simulink model "avr_simulation"  (R2021b)
settings: Solver=VariableStepAuto  StartTime=0.0  StopTime=1  RelTol=1e-3
undefined symbols (not defined in the file): E_1, E_2, initialOffset2, S_E_E1, S_E_E2, Ts
libraries: simulink x8, eeGeneralControl x6
settings Model: Creator=mouht  LastModifiedBy=mouht

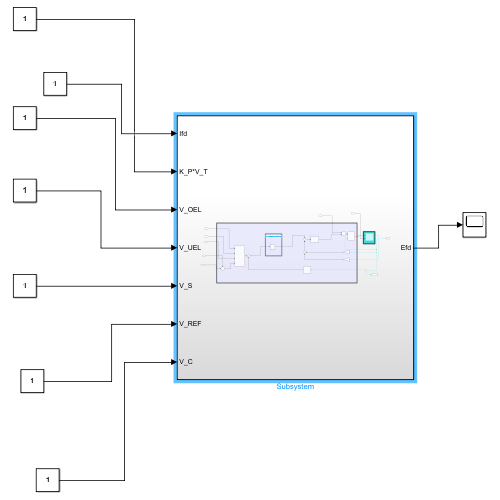
[thumbnail: Simulink's stored preview of the top-level diagram]
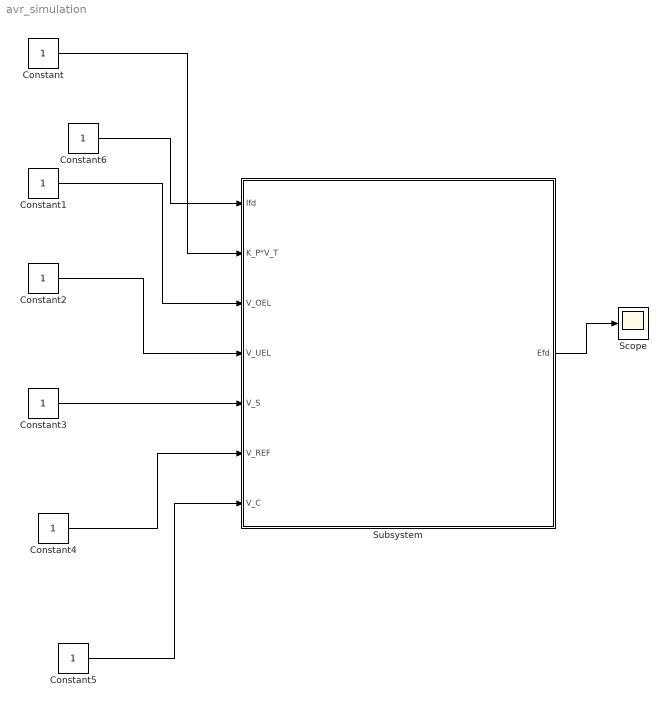
== system avr_simulation ==
  Constant{,1..6} (7 alike) : Constant
  Scope : Scope
  Subsystem : Subsystem
  wires:
  Constant5/1 -> Subsystem/7("V_C ")
  Constant4/1 -> Subsystem/6(V_REF)
  Constant3/1 -> Subsystem/5(V_S)
  Constant2/1 -> Subsystem/4(V_UEL)
  Constant1/1 -> Subsystem/3(V_OEL)
  Constant/1 -> Subsystem/2(K_P*V_T)
  Constant6/1 -> Subsystem/1(Ifd)
  Subsystem/1(Efd) -> Scope/1

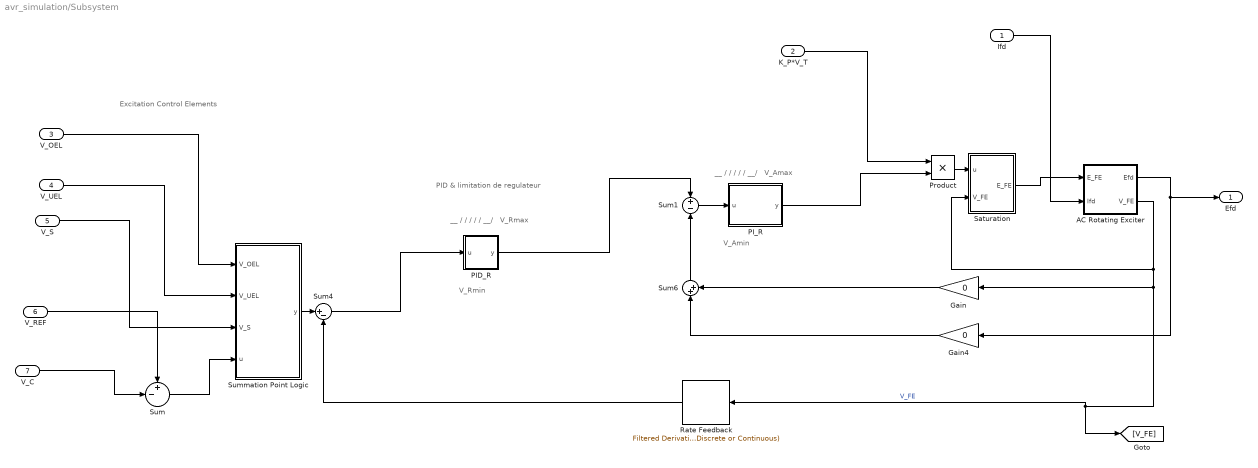
== system avr_simulation/Subsystem ==
  note: PID & limitation de regulateur
  note: __
      |               /
      |             /
      |           /
      |         /
      |       /
      | __/
  note: Excitation
      | Control
      | Elements
  note: V_Rmax
  note: V_Rmin
  note: __
      |               /
      |             /
      |           /
      |         /
      |       /
      | __/
  note: V_Amax
  note: V_Amin
  Ifd : Inport
  K_P*V_T : Inport  Port=2
  V_OEL : Inport  Port=3
  V_UEL : Inport  Port=4
  V_S : Inport  Port=5
  V_REF : Inport  Port=6
  "V_C " : Inport  Port=7
  AC Rotating Exciter : Subsystem
  Gain : Gain  Gain=0
  Gain4 : Gain  Gain=0
  PID_R : Subsystem
  PI_R : Subsystem
  Product : Product
  Rate Feedback : eeGeneralControl/Filtered Derivative (Discrete or Continuous)  K=0  T=1  B=inf  A=-inf  minRatio=10  init_option=Inherited from block input  x0=0  Ts=-1
      settings: SourceProductBaseCode=PS
  Saturation : Subsystem
  Sum : Sum  Inputs=+-|  InputSameDT=on  SaturateOnIntegerOverflow=on  OutDataTypeStr=Inherit: Same as first input
  Sum1 : Sum  Inputs=+-  InputSameDT=on  SaturateOnIntegerOverflow=on  OutDataTypeStr=Inherit: Same as first input
  Sum4 : Sum  Inputs=|+-  InputSameDT=on  SaturateOnIntegerOverflow=on  OutDataTypeStr=Inherit: Same as first input
  Sum6 : Sum  Inputs=|++  InputSameDT=on  SaturateOnIntegerOverflow=on  OutDataTypeStr=Inherit: Same as first input
  Summation Point Logic : Subsystem
  Efd : Outport
  wires:
  Product/1 -> Saturation/1(u)
  AC Rotating Exciter/2(V_FE) -> [V_FE], Rate Feedback/1, Gain/1, Saturation/2(V_FE)  "V_FE"
  Gain/1 -> Sum6/2
  Gain4/1 -> Sum6/1
  Saturation/1(E_FE) -> AC Rotating Exciter/1(E_FE)
  PI_R/1(y) -> Product/2
  V_S/1 -> Summation Point Logic/3(V_S)
  AC Rotating Exciter/1(Efd) -> Efd/1, Gain4/1
  Sum1/1 -> PI_R/1(u)
  Sum4/1 -> PID_R/1(u)
  Sum6/1 -> Sum1/2
  Sum/1 -> Summation Point Logic/4(u)
  PID_R/1(y) -> Sum1/1
  Rate Feedback/1 -> Sum4/2
  Summation Point Logic/1(y) -> Sum4/1
  K_P*V_T/1 -> Product/1
  V_OEL/1 -> Summation Point Logic/1(V_OEL)
  Ifd/1 -> AC Rotating Exciter/2(Ifd)
  V_REF/1 -> Sum/1
  "V_C "/1 -> Sum/2
  V_UEL/1 -> Summation Point Logic/2(V_UEL)

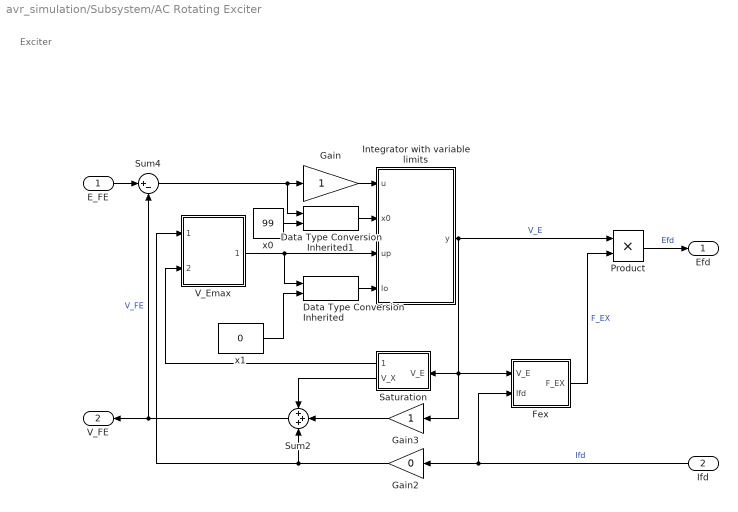
== system avr_simulation/Subsystem/AC Rotating Exciter ==
  note: Exciter
  E_FE : Inport
  Ifd : Inport  Port=2
  Data Type Conversion Inherited : simulink/Signal Attributes/Data Type Conversion Inherited  ConvertRealWorld=Real World Value  DoSatur=off
      settings: SourceProductBaseCode=SL
  Data Type Conversion Inherited1 : simulink/Signal Attributes/Data Type Conversion Inherited  ConvertRealWorld=Real World Value  DoSatur=off
      settings: SourceProductBaseCode=SL
  Fex : Subsystem  mask{K_C=0}
      mask prompts: K_C "Rectifier regulation factor, K_C (pu):"
  Gain : Gain  SaturateOnIntegerOverflow=on  OutDataTypeStr=Inherit: Same as input  ParamDataTypeStr=Inherit: Same as input
  Gain2 : Gain  Gain=0  SaturateOnIntegerOverflow=on  OutDataTypeStr=Inherit: Same as input  ParamDataTypeStr=Inherit: Same as input
  Gain3 : Gain  SaturateOnIntegerOverflow=on  OutDataTypeStr=Inherit: Same as input  ParamDataTypeStr=Inherit: Same as input
  Integrator with variable limits : Subsystem
  Product : Product  OutDataTypeStr=Inherit: Same as first input
  Saturation : Subsystem  mask{Ve21=[4.5 3.38], SeVe21=[1.36 1.5]}
      mask prompts: Ve21 "Field voltage values, [Ve2(pu) Ve1(pu)]:"; SeVe21 "Saturation values, [SeVe2(pu) SeVe1(pu)]:"
      mask init:
      | Ve2=Ve21(1);Ve1=Ve21(2);
      | SeVe2=SeVe21(1);SeVe1=SeVe21(2);
  Sum2 : Sum  Inputs=+++  InputSameDT=on  SaturateOnIntegerOverflow=on  OutDataTypeStr=Inherit: Same as first input
  Sum4 : Sum  Inputs=|+-  InputSameDT=on  SaturateOnIntegerOverflow=on  OutDataTypeStr=Inherit: Same as first input
  V_Emax : Subsystem
  x0 : Constant  Value=99
  x1 : Constant  Value=0
  Efd : Outport  VectorParamsAs1DForOutWhenUnconnected=off
  V_FE : Outport  Port=2  VectorParamsAs1DForOutWhenUnconnected=off
  wires:
  Gain2/1 -> V_Emax/1(Ifd*K_D), Sum2/3
  Fex/1(F_EX) -> Product/2  "F_EX"
  Product/1 -> Efd/1  "Efd"
  Gain3/1 -> Sum2/2
  Saturation/2(V_X) -> Sum2/1
  Sum4/1 -> Data Type Conversion Inherited1/1, Gain/1
  Gain/1 -> Integrator with variable limits/1(u)
  Integrator with variable limits/1(y) -> Gain3/1, Fex/1(V_E), Saturation/1(V_E), Product/1  "V_E"
  E_FE/1 -> Sum4/1
  Sum2/1 -> Sum4/2, V_FE/1  "V_FE"
  Ifd/1 -> Gain2/1, Fex/2(Ifd)  "Ifd"
  Saturation/1(S_E(V_E)) -> V_Emax/2(S_E(V_E))
  Data Type Conversion Inherited/1 -> Integrator with variable limits/4(lo)
  x1/1 -> Data Type Conversion Inherited/2
  V_Emax/1(V_Emax) -> Integrator with variable limits/3(up), Data Type Conversion Inherited/1
  Data Type Conversion Inherited1/1 -> Integrator with variable limits/2(x0)
  x0/1 -> Data Type Conversion Inherited1/2

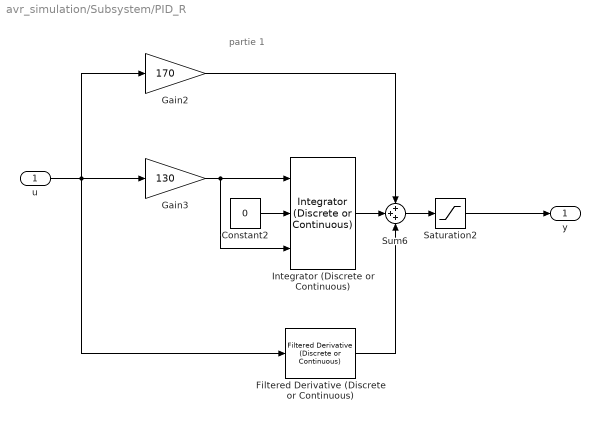
== system avr_simulation/Subsystem/PID_R ==
  note: partie 1
  u : Inport
  Constant2 : Constant  Value=0
  Filtered Derivative (Discrete or Continuous) : eeGeneralControl/Filtered Derivative (Discrete or Continuous)  K=0  T=1  B=inf  A=-inf  minRatio=10  init_option=Inherited from block input  x0=0  Ts=-1
      settings: SourceProductBaseCode=PS
  Gain2 : Gain  Gain=170
  Gain3 : Gain  Gain=130
  Integrator (Discrete or Continuous) : eeGeneralControl/Integrator (Discrete or Continuous)  LabelModeActiveChoice=Discrete  ExternalReset=level  LimitType=Anti-windup  B=10  A=0  Ts=-1
      settings: SourceProductBaseCode=PS
  Saturation2 : Saturate  UpperLimit=10  LowerLimit=0
  Sum6 : Sum  Inputs=+++
  y : Outport
  wires:
  Sum6/1 -> Saturation2/1
  Gain3/1 -> Integrator (Discrete or Continuous)/1, Integrator (Discrete or Continuous)/3
  u/1 -> Filtered Derivative (Discrete or Continuous)/1, Gain2/1, Gain3/1
  Constant2/1 -> Integrator (Discrete or Continuous)/2
  Integrator (Discrete or Continuous)/1 -> Sum6/2
  Gain2/1 -> Sum6/1
  Saturation2/1 -> y/1
  Filtered Derivative (Discrete or Continuous)/1 -> Sum6/3

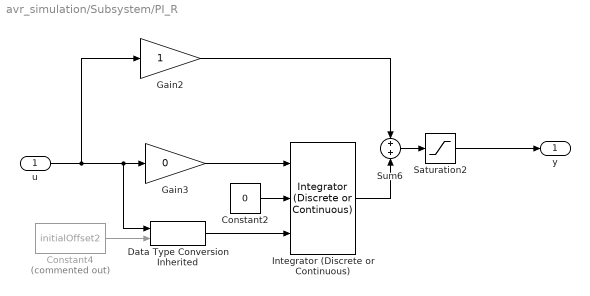
== system avr_simulation/Subsystem/PI_R ==
  u : Inport
  Constant2 : Constant  Value=0
  Constant4 : Constant  Commented=on  Value=initialOffset2
  Data Type Conversion Inherited : simulink/Signal Attributes/Data Type Conversion Inherited  ConvertRealWorld=Real World Value  DoSatur=off
      settings: SourceProductBaseCode=SL
  Gain2 : Gain
  Gain3 : Gain  Gain=0
  Integrator (Discrete or Continuous) : eeGeneralControl/Integrator (Discrete or Continuous)  LabelModeActiveChoice=Discrete  ExternalReset=level  LimitType=Anti-windup  B=10  A=0  Ts=-1
      settings: SourceProductBaseCode=PS
  Saturation2 : Saturate  UpperLimit=10  LowerLimit=0
  Sum6 : Sum
  y : Outport
  wires:
  Sum6/1 -> Saturation2/1
  Gain3/1 -> Integrator (Discrete or Continuous)/1
  u/1 -> Gain2/1, Data Type Conversion Inherited/1, Gain3/1
  Constant2/1 -> Integrator (Discrete or Continuous)/2
  Integrator (Discrete or Continuous)/1 -> Sum6/2
  Gain2/1 -> Sum6/1
  Saturation2/1 -> y/1
  Data Type Conversion Inherited/1 -> Integrator (Discrete or Continuous)/3
  Constant4/1 -> Data Type Conversion Inherited/2

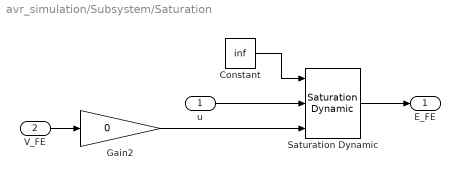
== system avr_simulation/Subsystem/Saturation ==
  u : Inport
  V_FE : Inport  Port=2
  Constant : Constant  Value=inf
  Gain2 : Gain  Gain=0
  Saturation Dynamic : simulink/Discontinuities/Saturation Dynamic  OutMin=[]  OutMax=[]  OutDataTypeStr=Inherit: Same as second input  OutDataType=fixdt(1, 16)  OutScaling=2^-10  DoSatur=off
  E_FE : Outport
  wires:
  Saturation Dynamic/1 -> E_FE/1
  u/1 -> Saturation Dynamic/2
  V_FE/1 -> Gain2/1
  Constant/1 -> Saturation Dynamic/1
  Gain2/1 -> Saturation Dynamic/3

== system avr_simulation/Subsystem/Summation Point Logic ==
  V_OEL : Inport
  V_UEL : Inport  Port=2
  V_S : Inport  Port=3  SampleTime=Ts
  u : Inport  Port=4
  Sum : Sum  Inputs=++++
  y : Outport  VectorParamsAs1DForOutWhenUnconnected=off
  wires:
  V_OEL/1 -> Sum/1
  V_UEL/1 -> Sum/2
  Sum/1 -> y/1
  u/1 -> Sum/4
  V_S/1 -> Sum/3

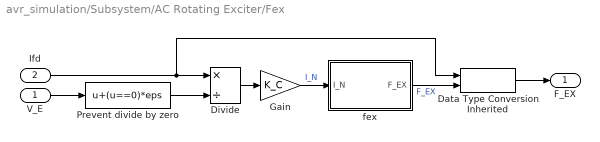
== system avr_simulation/Subsystem/AC Rotating Exciter/Fex ==
  V_E : Inport
  Ifd : Inport  Port=2
  Data Type Conversion Inherited : simulink/Signal Attributes/Data Type Conversion Inherited  ConvertRealWorld=Real World Value  DoSatur=off
      settings: SourceProductBaseCode=SL
  Divide : Product  Inputs=*/
  Gain : Gain  Gain=K_C  OutDataTypeStr=double
  Prevent divide by zero : Fcn  Expr=u+(u==0)*eps
  fex : MATLAB Function  TreatAsAtomicUnit=on
  F_EX : Outport  VectorParamsAs1DForOutWhenUnconnected=off
  wires:
  Gain/1 -> fex/1(I_N)  "I_N"
  Divide/1 -> Gain/1
  V_E/1 -> Prevent divide by zero/1
  Ifd/1 -> Data Type Conversion Inherited/1, Divide/1
  Prevent divide by zero/1 -> Divide/2
  fex/1(F_EX) -> Data Type Conversion Inherited/2  "F_EX"
  Data Type Conversion Inherited/1 -> F_EX/1

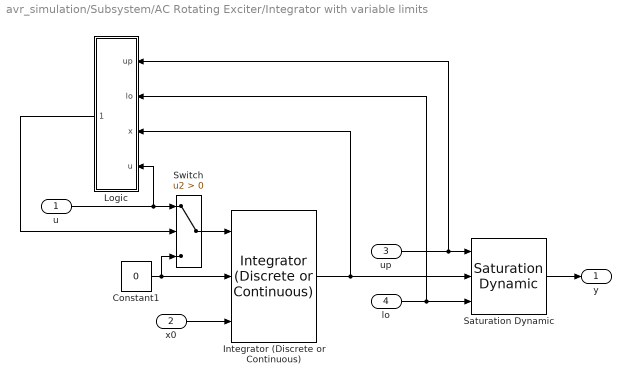
== system avr_simulation/Subsystem/AC Rotating Exciter/Integrator with variable limits ==
  u : Inport
  x0 : Inport  Port=2
  up : Inport  Port=3
  lo : Inport  Port=4
  Constant1 : Constant  Value=0
  Integrator (Discrete or Continuous) : eeGeneralControl/Integrator (Discrete or Continuous)  LabelModeActiveChoice=Discrete  ExternalReset=level  LimitType=Anti-windup  B=inf  A=-inf  Ts=-1
      settings: SourceProductBaseCode=PS
  Logic : Subsystem
  Saturation Dynamic : simulink/Discontinuities/Saturation Dynamic  OutMin=[]  OutMax=[]  OutDataTypeStr=Inherit: Same as second input  OutDataType=fixdt(1, 16)  OutScaling=2^-10  DoSatur=off
  Switch : Switch  Criteria=u2 > Threshold  OutDataTypeStr=Inherit: Same as first input
  y : Outport
  wires:
  up/1 -> Saturation Dynamic/1, Logic/1(up)
  Saturation Dynamic/1 -> y/1
  Switch/1 -> Integrator (Discrete or Continuous)/1
  lo/1 -> Saturation Dynamic/3, Logic/2(lo)
  u/1 -> Logic/4(u), Switch/1
  Constant1/1 -> Switch/3, Integrator (Discrete or Continuous)/2
  x0/1 -> Integrator (Discrete or Continuous)/3
  Integrator (Discrete or Continuous)/1 -> Logic/3(x), Saturation Dynamic/2
  Logic/1(Switch) -> Switch/2

== system avr_simulation/Subsystem/AC Rotating Exciter/Saturation ==
  V_E : Inport
  Product : Product  InputSameDT=on  RndMeth=Zero  SaturateOnIntegerOverflow=on  OutDataTypeStr=Inherit: Same as first input
  Saturation : Lookup_n-D  NumberOfTableDimensions=1  BreakpointsForDimension1=[0 E_2 E_1]  Table=[0 S_E_E2 S_E_E1]  InternalRulePriority=Speed  RndMeth=Simplest  InputSameDT=on
  S_E(V_E) : Outport  VectorParamsAs1DForOutWhenUnconnected=off
  V_X : Outport  Port=2  VectorParamsAs1DForOutWhenUnconnected=off
  wires:
  Product/1 -> V_X/1  "V_X"
  Saturation/1 -> Product/2, S_E(V_E)/1
  V_E/1 -> Product/1, Saturation/1

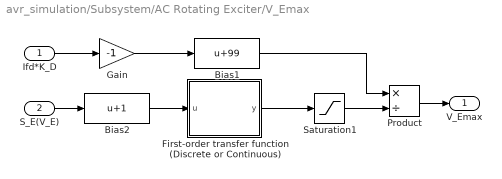
== system avr_simulation/Subsystem/AC Rotating Exciter/V_Emax ==
  Ifd*K_D : Inport
  S_E(V_E) : Inport  Port=2
  Bias1 : Bias  Bias=99
  Bias2 : Bias  Bias=1
  First-order transfer function (Discrete or Continuous) : Subsystem  mask(First-order transfer function (Discrete or Continuous)){T=1e-6, x0=1, Ts=-1}
      mask prompts: T "physmod:ee:library:comments:control:eeGeneralControl:TimeConstant_MP"; x0 "physmod:ee:library:comments:control:eeGeneralControl:InitialState_MP"; Ts "physmod:ee:library:comments:control:eeGeneralControl:SampleTime1ForInherited_MP"
      mask TypeOptions Ts:
      | Integrator
      | (Discrete or Continuous)/Ts
      mask DialogControl ParameterGroupVar Prompt: physmod:ee:library:comments:control:eeGeneralControl:tab_Parameters
      mask DialogControl T Prompt: Time constant
      mask DialogControl x0 Prompt: Initial state
      mask DialogControl Ts Prompt: Sample time (-1 for inherited)
      mask Display: dpoly(1,[T 1],'s');
  Gain : Gain  Gain=-1
  Product : Product  Inputs=*/
  Saturation1 : Saturate  UpperLimit=inf  LowerLimit=eps
  V_Emax : Outport
  wires:
  S_E(V_E)/1 -> Bias2/1
  Saturation1/1 -> Product/2
  Ifd*K_D/1 -> Gain/1
  Gain/1 -> Bias1/1
  Bias1/1 -> Product/1
  Product/1 -> V_Emax/1
  Bias2/1 -> First-order transfer function (Discrete or Continuous)/1(u)
  First-order transfer function (Discrete or Continuous)/1(y) -> Saturation1/1

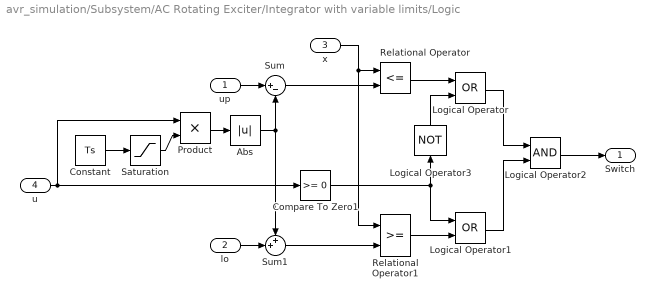
== system avr_simulation/Subsystem/AC Rotating Exciter/Integrator with variable limits/Logic ==
  up : Inport
  lo : Inport  Port=2
  x : Inport  Port=3
  u : Inport  Port=4
  Abs : Abs
  Compare To Zero1 : simulink/Logic and Bit Operations/Compare To Zero  relop=>=  OutDataTypeStr=uint8  ZeroCross=off
  Constant : Constant  Value=Ts
  Logical Operator : Logic  Operator=OR  AllPortsSameDT=off  OutDataTypeStr=boolean
  Logical Operator1 : Logic  Operator=OR  AllPortsSameDT=off  OutDataTypeStr=boolean
  Logical Operator2 : Logic  AllPortsSameDT=off  OutDataTypeStr=boolean
  Logical Operator3 : Logic  Operator=NOT  AllPortsSameDT=off  OutDataTypeStr=boolean
  Product : Product  OutDataTypeStr=Inherit: Same as first input
  Relational Operator : RelationalOperator  Operator=<=  OutDataTypeStr=boolean  RndMeth=Nearest
  Relational Operator1 : RelationalOperator  OutDataTypeStr=boolean  RndMeth=Nearest
  Saturation : Saturate  UpperLimit=inf  LowerLimit=0
  Sum : Sum  Inputs=|+-
  Sum1 : Sum  Inputs=++|
  Switch : Outport
  wires:
  Relational Operator1/1 -> Logical Operator1/2
  x/1 -> Relational Operator1/1, Relational Operator/1
  Logical Operator/1 -> Logical Operator2/1
  Relational Operator/1 -> Logical Operator/1
  u/1 -> Compare To Zero1/1, Product/1
  Compare To Zero1/1 -> Logical Operator1/1, Logical Operator3/1
  Logical Operator1/1 -> Logical Operator2/2
  Sum1/1 -> Relational Operator1/2
  lo/1 -> Sum1/2
  Sum/1 -> Relational Operator/2
  Abs/1 -> Sum/2, Sum1/1
  Constant/1 -> Saturation/1
  Product/1 -> Abs/1
  Logical Operator2/1 -> Switch/1
  up/1 -> Sum/1
  Logical Operator3/1 -> Logical Operator/2
  Saturation/1 -> Product/2

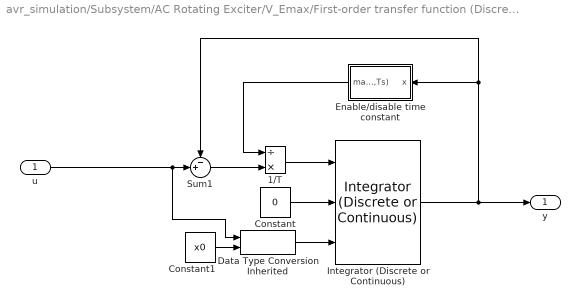
== system avr_simulation/Subsystem/AC Rotating Exciter/V_Emax/First-order transfer function (Discrete or Continuous) ==
  u : Inport
  1/T : Product  Inputs=/*
  Constant : Constant  Value=0
  Constant1 : Constant  Value=x0
  Data Type Conversion Inherited : simulink/Signal Attributes/Data Type Conversion Inherited  ConvertRealWorld=Real World Value  DoSatur=off
      settings: SourceProductBaseCode=SL
  Enable/disable time constant : Subsystem
  Integrator (Discrete or Continuous) : eeGeneralControl/Integrator (Discrete or Continuous)  LabelModeActiveChoice=Discrete  ExternalReset=level  LimitType=Anti-windup  B=inf  A=-inf  Ts=Ts
      settings: SourceProductBaseCode=PS
  Sum1 : Sum  Inputs=-+|
  y : Outport  VectorParamsAs1DForOutWhenUnconnected=off
  wires:
  u/1 -> Data Type Conversion Inherited/1, Sum1/2
  Sum1/1 -> 1/T/2
  1/T/1 -> Integrator (Discrete or Continuous)/1
  Enable/disable time constant/1(max(T,Ts)) -> 1/T/1
  Integrator (Discrete or Continuous)/1 -> Sum1/1, Enable/disable time constant/1(x), y/1
  Constant/1 -> Integrator (Discrete or Continuous)/2
  Constant1/1 -> Data Type Conversion Inherited/2
  Data Type Conversion Inherited/1 -> Integrator (Discrete or Continuous)/3

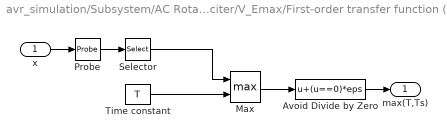
== system avr_simulation/Subsystem/AC Rotating Exciter/V_Emax/First-order transfer function (Discrete or Continuous)/Enable//disable time constant ==
  x : Inport
  Avoid Divide by Zero : Fcn  Expr=u+(u==0)*eps
  Max : MinMax  Function=max  Inputs=2  OutDataTypeStr=Inherit: Same as first input
  Probe : Probe  ProbeWidth=off  ProbeComplexSignal=off  ProbeSampleTimeDataType=Same as input
  Selector : Selector  InputPortWidth=2  IndexOptions=Index vector (dialog)  Indices=1  OutputSizes=1
  Time constant : Constant  Value=T  SampleTime=Ts
  max(T,Ts) : Outport  VectorParamsAs1DForOutWhenUnconnected=off
  wires:
  Max/1 -> Avoid Divide by Zero/1
  Probe/1 -> Selector/1
  Time constant/1 -> Max/2
  x/1 -> Probe/1
  Selector/1 -> Max/1
  Avoid Divide by Zero/1 -> max(T,Ts)/1

== matlab function avr_simulation/Subsystem/AC Rotating Exciter/Fex/fex ==
  data: I_N input; F_EX output
function F_EX = fex(I_N)
% AVRFEX Rectifier regulation characteristic based on: IEEE Recommended
% Practice for Excitation System Models for Power System Stability Studies,
% IEEE Std 421.5-2006,Annex D, Rectifier Regulation

F_EX = ee.control.sm.fex(I_N);

end
